simulink model "Bicycle_nonlinear"  (R2024b)
settings: Solver=VariableStepAuto  StartTime=0.0  StopTime=T  RelTol=1e-3
undefined symbols (not defined in the file): L, theta_i, x_i, y_i
libraries: robotmobilelib x1, sim3dlib x1, sim3dautolib x1
settings Model: Creator=loren  LastModifiedBy=loren

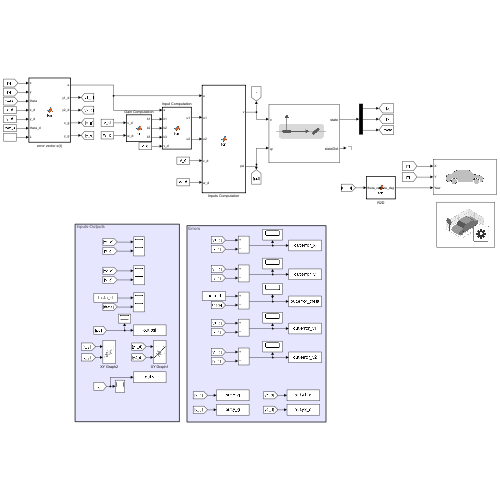
[thumbnail: Simulink's stored preview of the top-level diagram]
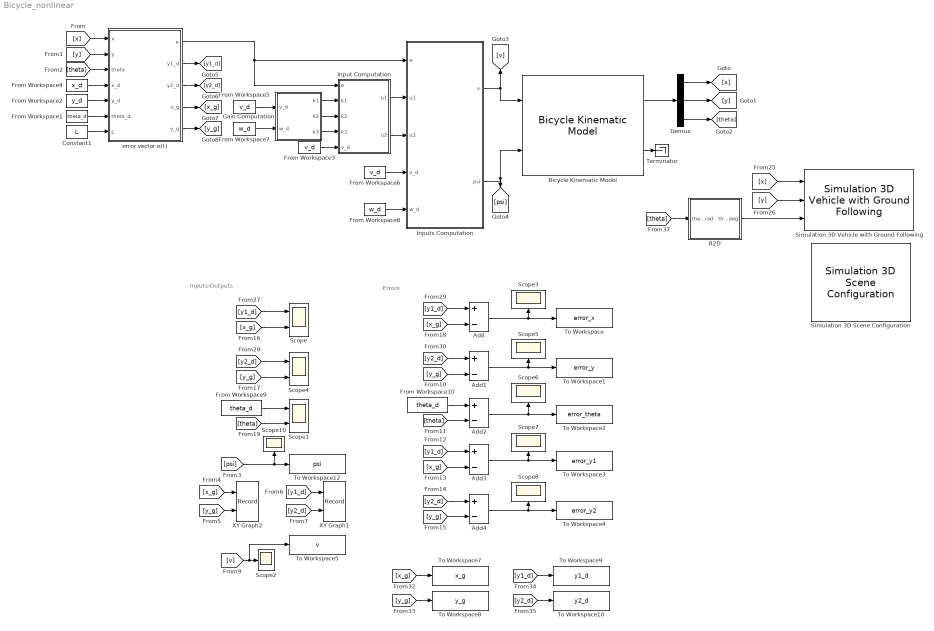
== system Bicycle_nonlinear ==
  note: Errors
  note: Inputs-Outputs
  Add{,1..4} (5 alike) : Sum  Inputs=+-
  Bicycle Kinematic Model : robotmobilelib/Bicycle Kinematic Model  VehicleInputs=Vehicle Speed & Steering Angle  WheelBase=L  VehicleSpeedRange=[-5, 5]  MaxSteeringAngle=pi/3  InitialState=q_i  SimulateUsing=Interpreted execution
  Constant1 : Constant  Value=L
  Demux : Demux  Outputs=3
  From Workspace1 : FromWorkspace  VariableName=theta_d
  From Workspace10 : FromWorkspace  VariableName=theta_d
  From Workspace2 : FromWorkspace  VariableName=y_d
  From Workspace3 : FromWorkspace  VariableName=v_d
  From Workspace4 : FromWorkspace  VariableName=x_d
  From Workspace5 : FromWorkspace  VariableName=v_d
  From Workspace6 : FromWorkspace  VariableName=v_d
  From Workspace7 : FromWorkspace  VariableName=w_d
  From Workspace8 : FromWorkspace  VariableName=w_d
  From Workspace9 : FromWorkspace  VariableName=theta_d
  Gain Computation : MATLAB Function  TreatAsAtomicUnit=on
  Input Computation : MATLAB Function  TreatAsAtomicUnit=on
  Inputs Computation : MATLAB Function  TreatAsAtomicUnit=on
  R2D : MATLAB Function  TreatAsAtomicUnit=on
  Scope : Scope  NumInputPorts=2
  Scope1 : Scope  NumInputPorts=2
  Scope{2..3,5..8,10} (7 alike) : Scope
  Scope4 : Scope  NumInputPorts=2
  Simulation 3D Scene Configuration : sim3dlib/Simulation 3D Scene Configuration  Priority=0  ProjectFormat=Default Scenes  SceneDesc=Open surface  ProjectName=C:\Program Files\MATLAB\R2024b\toolbox\shared\sim3d_projects\automotive_project_windows\UE\WindowsNoEditor\VehicleSimulation.exe  ScenePath=/Game/Maps/HwStrght  EnableOpenDRIVE=off  vehTagList={'Custom';'Scene Origin';'SimulinkVehicle1'}  vehTag=SimulinkVehicle1  FreeCameraInitialTranslation=[0, 0, 0]  FreeCameraDefaultInitialTranslation=[-6, 0, 2]  FreeCameraInitialRotation=[0, 0, 0]  FreeCameraDefaultInitialRotation=[0, -15, 0]  OpVisEn=off  Ts=.02  EnableWindow=on  EnableRemoteAccess=off  EnableWeather=off  SunAzimuth=90  SunAltitude=40.0  EnableGeospatialSun=off  Latitude=0  Longitude=0  Date=2023-01-01  Time=10:30:00  GeoTimeZone=-5.0  SunDaylightSaving=off  wind=1  clouds=10  EnableVolumetricClouds=off  CloudCoverage=0  CloudAltitude=6  fog=0  rain=0  RaindropsEffect=off  SnowDensity=0  EnableGeospatial=off  UseTrueOrigin=off  OriginHeight=200  OriginLatitude=40.744652  OriginLongitude=-73.988864  MapStyle=Aerial  AdditionalAssetIDs=[]  UseAdvancedSunSky=off  SolarTime=11  TimeZone=-5  Day=21  Month=9  Year=2022  UseDaylightSavingTime=on  DSTStartDay=10  DSTStartMonth=3  DSTEndDay=3  DSTEndMonth=11  DSTSwitchHour=2  sensorTag=MainCamera1  sensorId=1  sensorName=MainCamera1  mountLoc=Origin  offsetFlag=off  tmountOffset=[0, 0, 0]  rmountOffset=[0, 0, 0]  HorizontalResolution=1280  VerticalResolution=720  HorizontalFOV=60  mountPoint=[0 0 0]  mountOrientation=[0 0 0]  aMode=2  ID=1  GeoTrigger=Inactive
      settings: LibrarySourceBlock=vehdynlibsim3dcore/Simulation 3D Scene Configuration
  Simulation 3D Vehicle with Ground Following : sim3dautolib/Simulation 3D Vehicle with Ground Following  Priority=-1  PassVehMesh=Sedan  MeshPath=/MathWorksAutomotiveContent/Vehicles/Muscle/Meshes/SK_MuscleCar.SK_MuscleCar  TrackWidth=1.9  WheelBase=3  WheelRadius=0.35  VehColor=Black  InitialPos=[x_i, y_i, 0]  InitialRot=[0, 0, theta_i*180/pi]  ActorName=SimulinkVehicle1  SampleTime=0.01  ActorType=SimulinkVehicle  ID=1  aMode=3  ActorTag=SimulinkVehicle1  CoordinateScheme=ISO  VehLightsControl=off  HeadlightColor=[ 1, 1, 1 ]  HighBeamIntensity=100000  LowBeamIntensity=60000  HighBeamConeAngle=70  LowBeamConeAngle=70  LeftHeadlightOrientation=[ 0, 0 ]  RightHeadlightOrientation=[ 0, 0 ]  BrakelightIntensity=500  ReverselightIntensity=500  SignallightIntensity=500  SignallightPeriod=1  SignalPulseWidth=50  TransformOutportEnabled=off
      settings: LibrarySourceBlock=drivingsim3d/Simulation 3D Vehicle with Ground Following
  Terminator : Terminator
  To Workspace : ToWorkspace  VariableName=error_x  SaveFormat=Timeseries  SampleTime=-1
  To Workspace1 : ToWorkspace  VariableName=error_y  SaveFormat=Timeseries  SampleTime=-1
  To Workspace10 : ToWorkspace  VariableName=y2_d  SaveFormat=Timeseries  SampleTime=-1
  To Workspace12 : ToWorkspace  VariableName=psi  SaveFormat=Timeseries  SampleTime=-1
  To Workspace2 : ToWorkspace  VariableName=error_theta  SaveFormat=Timeseries  SampleTime=-1
  To Workspace3 : ToWorkspace  VariableName=error_y1  SaveFormat=Timeseries  SampleTime=-1
  To Workspace4 : ToWorkspace  VariableName=error_y2  SaveFormat=Timeseries  SampleTime=-1
  To Workspace5 : ToWorkspace  VariableName=v  SaveFormat=Timeseries  SampleTime=-1
  To Workspace7 : ToWorkspace  VariableName=x_g  SaveFormat=Timeseries  SampleTime=-1
  To Workspace8 : ToWorkspace  VariableName=y_g  SaveFormat=Timeseries  SampleTime=-1
  To Workspace9 : ToWorkspace  VariableName=y1_d  SaveFormat=Timeseries  SampleTime=-1
  XY Graph1 : Record  FileSettingsInternal="{\"entries\":[{\"content\":{\"excelSettings\":{\"content\":{},\"type\":\"Streamout.ExcelSettings\"}},\"type\":\"Streamout.FileSettingStorage\",\"uuid\":\"\"}],\"packageUris\":[\"http:\\/\\/schema.mathworks.com\\/mf0\\/streamout_blocks\\/R2020a\"],\"version\":\"1.0\"}"  Layout=[1 1]  SignalsInternal="{\"entries\":[{\"content\":{\"signals\":[{\"content\":{\"blockPath\":[],\"dimensions\":[1],\"domain\":\"\",\"lineColor\":\"#ff6929\",\"lineWidth\":2,\"port\":1,\"sid\":[\"\"],\"signalID\":1,\"signalName\":\"From6\"},\"type\":\"RecordBlkView.Signal\",\"uuid\":\"\"},{\"content\":{\"blockPath\":[],\"dimensions\":[1],\"domain\":\"\",\"lineColor\":\"#b746ff\",\"lineWidth\":2,\"port\":2,\"sid\":[\"\"],\"signalID\":2,\"signalName\":\"From7\"},\"type\":\"RecordBlkView.Signal\",\"uuid\":\"\"}]},\"type\":\"RecordBlkView.InputSignals\",\"uuid\":\"\"}],\"packageUris\":[\"http:\\/\\/schema.mathworks.com\\/mf0\\/streamout_blocks\\/R2020a\"],\"version\":\"1.0\"}"  VisualizationBindings="{\"xyplotplugin\":{\"info\":[{\"series\":[],\"subplotID\":1}]}}"  CompatibilityTag=XY
  XY Graph2 : Record  FileSettingsInternal="{\"entries\":[{\"content\":{\"excelSettings\":{\"content\":{},\"type\":\"Streamout.ExcelSettings\"}},\"type\":\"Streamout.FileSettingStorage\",\"uuid\":\"\"}],\"packageUris\":[\"http:\\/\\/schema.mathworks.com\\/mf0\\/streamout_blocks\\/R2020a\"],\"version\":\"1.0\"}"  Layout=[1 1]  SignalsInternal="{\"entries\":[{\"content\":{\"signals\":[{\"content\":{\"blockPath\":[],\"dimensions\":[1],\"domain\":\"\",\"lineColor\":\"#64d413\",\"lineWidth\":2,\"port\":1,\"sid\":[\"\"],\"signalID\":1,\"signalName\":\"From4\"},\"type\":\"RecordBlkView.Signal\",\"uuid\":\"\"},{\"content\":{\"blockPath\":[],\"dimensions\":[1],\"domain\":\"\",\"lineColor\":\"#ff13a6\",\"lineWidth\":2,\"port\":2,\"sid\":[\"\"],\"signalID\":2,\"signalName\":\"From5\"},\"type\":\"RecordBlkView.Signal\",\"uuid\":\"\"}]},\"type\":\"RecordBlkView.InputSignals\",\"uuid\":\"\"}],\"packageUris\":[\"http:\\/\\/schema.mathworks.com\\/mf0\\/streamout_blocks\\/R2020a\"],\"version\":\"1.0\"}"  VisualizationBindings="{\"xyplotplugin\":{\"info\":[{\"series\":[],\"subplotID\":1}]}}"  CompatibilityTag=XY
  error vector e(t) : MATLAB Function  TreatAsAtomicUnit=on
  wires:
  Bicycle Kinematic Model/2 -> Terminator/1
  Demux/1 -> [x]
  Inputs Computation/2(psi) -> Bicycle Kinematic Model/2, [psi]
  Inputs Computation/1(v) -> [v], Bicycle Kinematic Model/1
  From Workspace8/1 -> Inputs Computation/5(w_d)
  error vector e(t)/1(e) -> Input Computation/1(e), Inputs Computation/1(e)
  From Workspace6/1 -> Inputs Computation/4(v_d)
  Demux/3 -> [theta]
  Bicycle Kinematic Model/1 -> Demux/1
  From Workspace3/1 -> Input Computation/5(v_d)
  Demux/2 -> [y]
  Input Computation/1(u1) -> Inputs Computation/2(u1)
  Input Computation/2(u2) -> Inputs Computation/3(u2)
  Gain Computation/1(k1) -> Input Computation/2(k1)
  Gain Computation/3(k3) -> Input Computation/4(k3)
  Gain Computation/2(k2) -> Input Computation/3(k2)
  [x] -> error vector e(t)/1(x)
  [theta] -> error vector e(t)/3(theta)
  Constant1/1 -> error vector e(t)/7(L)
  [y] -> error vector e(t)/2(y)
  From Workspace2/1 -> error vector e(t)/5(y_d)
  From Workspace1/1 -> error vector e(t)/6(theta_d)
  From Workspace4/1 -> error vector e(t)/4(x_d)
  error vector e(t)/2(y1_d) -> [y1_d]
  error vector e(t)/3(y2_d) -> [y2_d]
  error vector e(t)/4(x_g) -> [x_g]
  error vector e(t)/5(y_g) -> [y_g]
  From Workspace7/1 -> Gain Computation/2(w_d)
  From Workspace5/1 -> Gain Computation/1(v_d)
  [y2_d] -> Scope4/1
  [y2_d] -> Add1/1
  Add1/1 -> Scope5/1, To Workspace1/1
  Add2/1 -> Scope6/1, To Workspace2/1
  [y_g] -> Add1/2
  [x_g] -> To Workspace7/1
  [y2_d] -> Add4/1
  [theta] -> Scope1/2
  [v] -> Scope2/1, To Workspace5/1
  Add/1 -> Scope3/1, To Workspace/1
  [x_g] -> Scope/2
  Add4/1 -> Scope8/1, To Workspace4/1
  [y1_d] -> Add3/1
  [y1_d] -> To Workspace9/1
  Add3/1 -> Scope7/1, To Workspace3/1
  [x_g] -> Add/2
  [y1_d] -> Add/1
  [y_g] -> XY Graph2/2
  [y_g] -> To Workspace8/1
  [x_g] -> XY Graph2/1
  From Workspace9/1 -> Scope1/1
  [y1_d] -> Scope/1
  [theta] -> Add2/2
  [psi] -> Scope10/1, To Workspace12/1
  [y1_d] -> XY Graph1/1
  [y2_d] -> To Workspace10/1
  [y_g] -> Add4/2
  [y2_d] -> XY Graph1/2
  [y_g] -> Scope4/2
  [x_g] -> Add3/2
  From Workspace10/1 -> Add2/1
  R2D/1(theta_deg) -> Simulation 3D Vehicle with Ground Following/3
  [x] -> Simulation 3D Vehicle with Ground Following/1
  [theta] -> R2D/1(theta_rad)
  [y] -> Simulation 3D Vehicle with Ground Following/2

== matlab function Bicycle_nonlinear/R2D ==
  data: theta_rad input; theta_deg output
function theta_deg = fcn(theta_rad)

theta_deg = theta_rad*180/pi;

== matlab function Bicycle_nonlinear/Gain Computation ==
  data: v_d input; k1 output; w_d input; k2 output; k3 output
function [k1, k2, k3] = fcn(v_d, w_d)

k1 = 0.05*(sqrt(v_d^2+w_d^2)); % k1(vd(t),wd(t))>0 bounded positive gain function
k2 = 0.005; % k2>0
k3 = 0.1*(abs(v_d) + abs(w_d)); % k3(vd(t),wd(t))>0 bounded positive gain function

== matlab function Bicycle_nonlinear/Input Computation ==
  data: e input; u1 output; k1 input; k2 input; k3 input; u2 output; v_d input
function [u1, u2] = fcn(e, k1, k2, k3, v_d)

u1 = -k1*e(1);
u2 = -k2*v_d*sin(e(3))/e(3)*e(2) - k3*e(3);

== matlab function Bicycle_nonlinear/Inputs Computation ==
  data: e input; v output; u1 input; u2 input; v_d input; w_d input; psi output
function [v, psi] = fcn(e, u1, u2, v_d, w_d)

L = 3.5;

v = v_d * cos(e(3)) - u1;
w = w_d - u2;

    if abs(v) > 1e-6  % Avoid singularity
        psi = atan((w * L) / v);
    else
        psi = 0;
    end

% Maximum feasible limit for psi
psi_max = 60 * pi/180;  % ±60 degrees
psi = max(-psi_max, min(psi_max, psi));

== matlab function Bicycle_nonlinear/error vector e(t) ==
  data: x input; e output; y input; theta input; x_d input; y_d input; theta_d input; L input; y1_d output; y2_d output; x_g output; y_g output
function [e, y1_d, y2_d, x_g, y_g] = fcn(x, y, theta, x_d, y_d, theta_d, L)

M = [ cos(theta), sin(theta), 0;
     -sin(theta), cos(theta), 0;
               0,          0, 1];

y1_d = x_d + (L/2) * cos(theta_d);
y2_d = y_d + (L/2) * sin(theta_d);

x_g = x + L/2 * cos(theta);
y_g = y + L/2 * sin(theta);

e_star = [y1_d - x_g; y2_d - y_g; theta_d - theta];
e = M * e_star;
